simulink model "Prismatic_Inverted_Pendulum"  (R2020b)
settings: Solver=VariableStepAuto  StartTime=0.0  StopTime=50  RelTol=1e-3
libraries: fuzblock x1
settings Model: Creator=Taha  LastModifiedBy=Taha

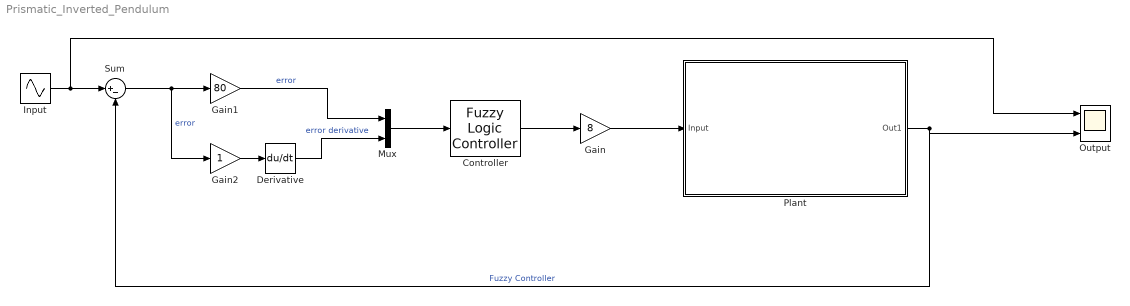
== system Prismatic_Inverted_Pendulum ==
  Controller : fuzblock/Fuzzy Logic  Controller  FIS="\"Inverted_Pendulum.fis\""  OutputSampleNumber=101  DataType=double  FuzzifiedInputs=off  RuleFiringStrengths=off  RuleOutputs=off  AggregatedOutputs=off  SimulateUsing=Interpreted execution  OutOfRangeInputValueMessage=warning  NoRuleFiredMessage=warning  EmptyOutputFuzzySetMessage=warning
  Derivative : Derivative
  Gain : Gain  Gain=8
  Gain1 : Gain  Gain=80
  Gain2 : Gain
  Input : Sin  Amplitude=0.1  Frequency=0.2  SampleTime=0
  Mux : Mux  Inputs=2
  Output : Scope  NumInputPorts=2
  Plant : Subsystem
      mask Display: image('The-inverted-pendulum-on-a-cart-system.png'); % Use "Edit Image" on toolstrip to change.
  Sum : Sum  Inputs=|+-
  wires:
  Plant/1(Out1) -> Output/2, Sum/2  "Fuzzy Controller"
  Controller/1 -> Gain/1
  Gain/1 -> Plant/1(Input)
  Input/1 -> Output/1, Sum/1
  Sum/1 -> Gain2/1, Gain1/1  "error"
  Mux/1 -> Controller/1
  Gain1/1 -> Mux/1  "error"
  Gain2/1 -> Derivative/1
  Derivative/1 -> Mux/2  "error derivative"

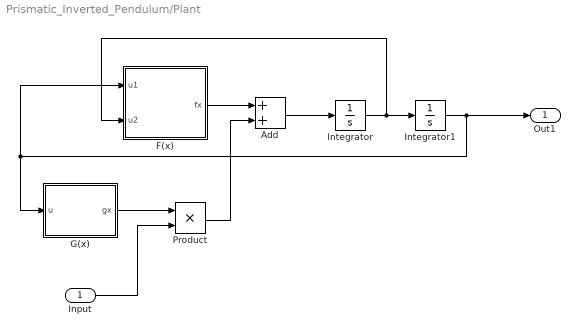
== system Prismatic_Inverted_Pendulum/Plant ==
  Input : Inport
  Add : Sum
  F(x) : MATLAB Function  TreatAsAtomicUnit=on
  G(x) : MATLAB Function  TreatAsAtomicUnit=on
  Integrator : Integrator
  Integrator1 : Integrator
  Product : Product
  Out1 : Outport
  wires:
  F(x)/1(fx) -> Add/1
  Integrator1/1 -> G(x)/1(u), F(x)/1(u1), Out1/1
  Product/1 -> Add/2
  G(x)/1(gx) -> Product/1
  Integrator/1 -> F(x)/2(u2), Integrator1/1
  Input/1 -> Product/2
  Add/1 -> Integrator/1

== matlab function Prismatic_Inverted_Pendulum/Plant/G(x) ==
  data: u input; gx output
function gx = compute_gx(u)
    % Inputs:
    % u  - State vector [u(1): angle (theta)]
    % mc - Mass of the cart [kg]
    % mp - Mass of the pendulum [kg]
    % lp - Length of the pendulum [m]
    mc = 0.1;
    mp = 1;
    lp = 0.5; 
    % Calculate gx based on the given equation
    numerator = cos(u(1)) / (mc + mp);
    denominator = lp * ((4/3) - (mp * cos(u(1))^2) / (mc + mp));
    gx = numerator / denominator;
end

== matlab function Prismatic_Inverted_Pendulum/Plant/F(x) ==
  data: u1 input; fx output; u2 input
function fx = compute_fx(u1,u2)
    % Inputs:
    % u  - State vector [u(1): angle (theta), u(2): angular velocity (omega)]
    % mc - Mass of the cart [kg]
    % mp - Mass of the pendulum [kg]
    % lp - Length of the pendulum [m]
    % g  - Gravitational acceleration [m/s^2]
    mc = 0.1;
    mp = 1;
    g = 9.8;
    lp = 0.5; 
    % Calculate fx based on the given equation
  fx= (g * sin(u1) - mp * lp * ((u2)^2) * cos(u1) * sin(u1)) / (lp * ((4/3) - (mp * cos(u1)^2) / (mc + mp)));
    
   
end
